simulink model "l7sim4"  (R2022b)
settings: Solver=VariableStepAuto  StartTime=0.0  StopTime=10.0  RelTol=1e-3
values from neighbouring files (symbols this model uses):
  T = 6')    [ex2l3.m]    (also in l7ex4.m = 0.01)
settings Model: Creator=gokuz  LastModifiedBy=gokuz

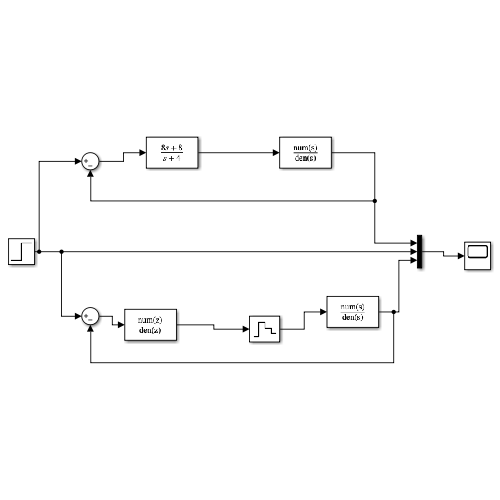
[thumbnail: Simulink's stored preview of the top-level diagram]
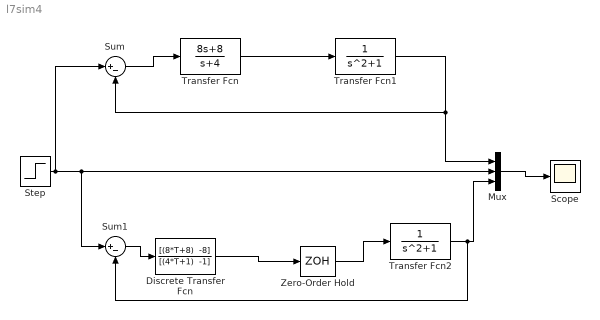
== system l7sim4 ==
  Discrete Transfer Fcn : DiscreteTransferFcn  Numerator="[(8*T+8)  -8]"  Denominator="[(4*T+1)  -1]"  InitialStates=1  SampleTime=T
  Mux : Mux  Inputs=3
  Scope : Scope
  Step : Step  SampleTime=0
  Sum : Sum  Inputs=|+-
  Sum1 : Sum  Inputs=|+-
  Transfer Fcn : TransferFcn  Numerator=[8 8]  Denominator="[1  4]"
  Transfer Fcn1 : TransferFcn  Denominator=[1 0 1]
  Transfer Fcn2 : TransferFcn  Denominator=[1 0 1]
  Zero-Order Hold : ZeroOrderHold  SampleTime=T
  wires:
  Mux/1 -> Scope/1
  Sum1/1 -> Discrete Transfer Fcn/1
  Step/1 -> Sum/1, Sum1/1, Mux/2
  Sum/1 -> Transfer Fcn/1
  Transfer Fcn/1 -> Transfer Fcn1/1
  Discrete Transfer Fcn/1 -> Zero-Order Hold/1
  Zero-Order Hold/1 -> Transfer Fcn2/1
  Transfer Fcn1/1 -> Sum/2, Mux/1
  Transfer Fcn2/1 -> Sum1/2, Mux/3
